simulink model "MotionLab"  (R2024a)
settings: Solver=VariableStepAuto  StartTime=0.0  StopTime=20  RelTol=1e-3  AbsTol=1e-3
values from neighbouring files (symbols this model uses):
  AmplitudeHeave = 0    [HMIVars.m]
  AmplitudePitch = 0    [HMIVars.m]
  AmplitudeRoll = 0    [HMIVars.m]
  AmplitudeSurge = 0    [HMIVars.m]
  AmplitudeSway = 0    [HMIVars.m]
  AmplitudeYaw = 0    [HMIVars.m]
  FrequencyHeave = 0    [HMIVars.m]
  FrequencyPitch = 0    [HMIVars.m]
  FrequencyRoll = 0    [HMIVars.m]
  FrequencySurge = 0    [HMIVars.m]
  FrequencySway = 0    [HMIVars.m]
  FrequencyYaw = 0    [HMIVars.m]
  OffsetHeave = 0    [HMIVars.m]
  OffsetPitch = 0    [HMIVars.m]
  OffsetRoll = 0    [HMIVars.m]
  OffsetSurge = 0    [HMIVars.m]
  OffsetSway = 0    [HMIVars.m]
  OffsetYaw = 0    [HMIVars.m]
  PhaseHeave = 0    [HMIVars.m]
  PhasePitch = 0    [HMIVars.m]
  PhaseRoll = 0    [HMIVars.m]
  PhaseSurge = 0    [HMIVars.m]
  PhaseSway = 0    [HMIVars.m]
  PhaseYaw = 0    [HMIVars.m]
undefined symbols (not defined in the file or in its folder): smiData, smiDataBig, smiDataBigTop, smiDataRobot, Var, X, Y, Z
libraries: sm_lib x438, nesl_utility x74
(part 14 of 14)

== system MotionLab/VHT eMotion-8000 Stewart Platform/UiA Stewart Platform/Top Platform/x3_134056_CARDAN_STEUN_stp_2_RIGID ==
  ReferenceFrame : sm_lib/Frames and Transforms/Reference Frame
  Solid : sm_lib/Body Elements/File Solid  ExtGeomFileName=.\CAD_Store\3-134056_CARDAN_STEUN.stp_Default_sldprt.STEP  UnitType=FromFile  ExtGeomFileUnits=m  StepReaderType=HEX  ExportConvexHullGeometry=off  InertiaType=Custom  BasedOnType=DensityFromFile  Density=1000  DensityUnits=kg/m^3  Mass=smiDataBig.Solid(7).mass  MassUnits=kg  CenterOfMass=smiDataBig.Solid(7).CoM  CenterOfMassUnits=mm  MomentsOfInertia=smiDataBig.Solid(7).MoI  MomentsOfInertiaUnits=kg*mm^2  ProductsOfInertia=smiDataBig.Solid(7).PoI  ProductsOfInertiaUnits=kg*mm^2  GraphicType=FromGeometry  MarkerShape=Sphere  MarkerSize=10  GraphicVisPropType=SimpleVisualProperties  GraphicDiffuseColor=smiDataBig.Solid(7).color  GraphicOpacity=smiDataBig.Solid(7).opacity  GraphicSpecularColor=[0.5 0.5 0.5 1.0]  GraphicAmbientColor=[0.15 0.15 0.15 1.0]  GraphicEmissiveColor=[0.0 0.0 0.0 1.0]  GraphicShininess=75  DoExposeReferenceFrame=on  SerializedFrames=<Frames><Frame><Id>Frame1</Id><Value><Name>F1</Name><Origin><Source>GeometricFeature</Source><FeatureName>cylindrical surface 89</FeatureName></Origin><PrimaryAxis><DefinedDirection>-Y</DefinedDirection><Source>ReferenceFrame</Source><SourceDirection>+Z</SourceDirection><FeatureName></FeatureName></PrimaryAxis><SecondaryAxis><DefinedDirection>+X</DefinedDirection><Source>ReferenceFrame</Source><SourceDirection>+X</SourceDirection><FeatureName></FeatureName></SecondaryAxis></Value></Frame><Frame><Id>Frame2</Id><Value><Name>F2</Name><Origin><Source>GeometricFeature</Source><FeatureName>cylindrical surface 83</FeatureName></Origin><PrimaryAxis><DefinedDirection>-Y</DefinedDirection><Source>ReferenceFrame</Source><SourceDirection>+Z</SourceDirection><FeatureName></FeatureName></PrimaryAxis><SecondaryAxis><DefinedDirection>+X</DefinedDirection><Source>ReferenceFrame</Source><SourceDirection>+X</SourceDirection><FeatureName></FeatureName></SecondaryAxis></Value></Frame><Frame><Id>Frame3</Id><Value><Name>F3</Name><Origin><Source>GeometricFeature</Source><FeatureName>planar surface 25</FeatureName></Origin><PrimaryAxis><DefinedDirection>+Z</DefinedDirection><Source>ReferenceFrame</Source><SourceDirection>+Z</SourceDirection><FeatureName></FeatureName></PrimaryAxis><SecondaryAxis><DefinedDirection>+X</DefinedDirection><Source>ReferenceFrame</Source><SourceDirection>+X</SourceDirection><FeatureName></FeatureName></SecondaryAxis></Value></Frame></Frames>
  F : PMIOPort  Side=Left
  F1 : PMIOPort  Port=2  Side=Right
  F2 : PMIOPort  Port=3  Side=Right
  connections:
  Solid/LConn1 -- F1/RConn1
  Solid/RConn2 -- ReferenceFrame/RConn1 -- F/RConn1
  Solid/LConn2 -- F2/RConn1

== system MotionLab/VHT eMotion-8000 Stewart Platform/UiA Stewart Platform/Top Platform/x3_134056_CARDAN_STEUN_stp_3_RIGID ==
  ReferenceFrame : sm_lib/Frames and Transforms/Reference Frame
  Solid : sm_lib/Body Elements/File Solid  ExtGeomFileName=.\CAD_Store\3-134056_CARDAN_STEUN.stp_Default_sldprt.STEP  UnitType=FromFile  ExtGeomFileUnits=m  StepReaderType=HEX  ExportConvexHullGeometry=off  InertiaType=Custom  BasedOnType=DensityFromFile  Density=1000  DensityUnits=kg/m^3  Mass=smiDataBig.Solid(7).mass  MassUnits=kg  CenterOfMass=smiDataBig.Solid(7).CoM  CenterOfMassUnits=mm  MomentsOfInertia=smiDataBig.Solid(7).MoI  MomentsOfInertiaUnits=kg*mm^2  ProductsOfInertia=smiDataBig.Solid(7).PoI  ProductsOfInertiaUnits=kg*mm^2  GraphicType=FromGeometry  MarkerShape=Sphere  MarkerSize=10  GraphicVisPropType=SimpleVisualProperties  GraphicDiffuseColor=smiDataBig.Solid(7).color  GraphicOpacity=smiDataBig.Solid(7).opacity  GraphicSpecularColor=[0.5 0.5 0.5 1.0]  GraphicAmbientColor=[0.15 0.15 0.15 1.0]  GraphicEmissiveColor=[0.0 0.0 0.0 1.0]  GraphicShininess=75  DoExposeReferenceFrame=on  SerializedFrames=<Frames><Frame><Id>Frame1</Id><Value><Name>F1</Name><Origin><Source>GeometricFeature</Source><FeatureName>cylindrical surface 89</FeatureName></Origin><PrimaryAxis><DefinedDirection>-Y</DefinedDirection><Source>ReferenceFrame</Source><SourceDirection>+Z</SourceDirection><FeatureName></FeatureName></PrimaryAxis><SecondaryAxis><DefinedDirection>+X</DefinedDirection><Source>ReferenceFrame</Source><SourceDirection>+X</SourceDirection><FeatureName></FeatureName></SecondaryAxis></Value></Frame><Frame><Id>Frame2</Id><Value><Name>F2</Name><Origin><Source>GeometricFeature</Source><FeatureName>cylindrical surface 83</FeatureName></Origin><PrimaryAxis><DefinedDirection>-Y</DefinedDirection><Source>ReferenceFrame</Source><SourceDirection>+Z</SourceDirection><FeatureName></FeatureName></PrimaryAxis><SecondaryAxis><DefinedDirection>+X</DefinedDirection><Source>ReferenceFrame</Source><SourceDirection>+X</SourceDirection><FeatureName></FeatureName></SecondaryAxis></Value></Frame><Frame><Id>Frame3</Id><Value><Name>F3</Name><Origin><Source>GeometricFeature</Source><FeatureName>planar surface 25</FeatureName></Origin><PrimaryAxis><DefinedDirection>+Z</DefinedDirection><Source>ReferenceFrame</Source><SourceDirection>+Z</SourceDirection><FeatureName></FeatureName></PrimaryAxis><SecondaryAxis><DefinedDirection>+X</DefinedDirection><Source>ReferenceFrame</Source><SourceDirection>+X</SourceDirection><FeatureName></FeatureName></SecondaryAxis></Value></Frame></Frames>
  F : PMIOPort  Side=Left
  F1 : PMIOPort  Port=2  Side=Right
  F2 : PMIOPort  Port=3  Side=Right
  connections:
  Solid/LConn2 -- F2/RConn1
  Solid/LConn1 -- F1/RConn1
  Solid/RConn2 -- ReferenceFrame/RConn1 -- F/RConn1

== system MotionLab/VHT eMotion-8000 Stewart Platform/UiA Stewart Platform/BaseFrame/x03_21_1320_ADM_Lower_Cardan_Baseplate_stp_1_RIGID/x03_21_1320_PDM_Base_Plate_stp_1_RIGID ==
  ReferenceFrame : sm_lib/Frames and Transforms/Reference Frame
  Solid : sm_lib/Body Elements/File Solid  ExtGeomFileName=.\CAD_Store\03-21-1320-PDM-Base Plate.stp_Default_sldprt.STEP  UnitType=FromFile  ExtGeomFileUnits=m  StepReaderType=HEX  ExportConvexHullGeometry=off  InertiaType=Custom  BasedOnType=DensityFromFile  Density=1000  DensityUnits=kg/m^3  Mass=smiDataBig.Solid(5).mass  MassUnits=kg  CenterOfMass=smiDataBig.Solid(5).CoM  CenterOfMassUnits=mm  MomentsOfInertia=smiDataBig.Solid(5).MoI  MomentsOfInertiaUnits=kg*mm^2  ProductsOfInertia=smiDataBig.Solid(5).PoI  ProductsOfInertiaUnits=kg*mm^2  GraphicType=FromGeometry  MarkerShape=Sphere  MarkerSize=10  GraphicVisPropType=SimpleVisualProperties  GraphicDiffuseColor=smiDataBig.Solid(5).color  GraphicOpacity=smiDataBig.Solid(5).opacity  GraphicSpecularColor=[0.5 0.5 0.5 1.0]  GraphicAmbientColor=[0.15 0.15 0.15 1.0]  GraphicEmissiveColor=[0.0 0.0 0.0 1.0]  GraphicShininess=75  DoExposeReferenceFrame=on  SerializedFrames=<Frames/>
  F : PMIOPort  Side=Left
  connections:
  ReferenceFrame/RConn1 -- Solid/RConn1 -- F/RConn1

== system MotionLab/VHT eMotion-8000 Stewart Platform/UiA Stewart Platform/BaseFrame/x03_21_1320_ADM_Lower_Cardan_Baseplate_stp_1_RIGID/x03_21_1320_PDM_Midplate_stp_1_RIGID ==
  ReferenceFrame : sm_lib/Frames and Transforms/Reference Frame
  Solid : sm_lib/Body Elements/File Solid  ExtGeomFileName=.\CAD_Store\03-21-1320-PDM-Midplate.stp_Default_sldprt.STEP  UnitType=FromFile  ExtGeomFileUnits=m  StepReaderType=HEX  ExportConvexHullGeometry=off  InertiaType=Custom  BasedOnType=DensityFromFile  Density=1000  DensityUnits=kg/m^3  Mass=smiDataBig.Solid(6).mass  MassUnits=kg  CenterOfMass=smiDataBig.Solid(6).CoM  CenterOfMassUnits=mm  MomentsOfInertia=smiDataBig.Solid(6).MoI  MomentsOfInertiaUnits=kg*mm^2  ProductsOfInertia=smiDataBig.Solid(6).PoI  ProductsOfInertiaUnits=kg*mm^2  GraphicType=FromGeometry  MarkerShape=Sphere  MarkerSize=10  GraphicVisPropType=SimpleVisualProperties  GraphicDiffuseColor=smiDataBig.Solid(6).color  GraphicOpacity=smiDataBig.Solid(6).opacity  GraphicSpecularColor=[0.5 0.5 0.5 1.0]  GraphicAmbientColor=[0.15 0.15 0.15 1.0]  GraphicEmissiveColor=[0.0 0.0 0.0 1.0]  GraphicShininess=75  DoExposeReferenceFrame=on  SerializedFrames=<Frames/>
  F : PMIOPort  Side=Left
  connections:
  ReferenceFrame/RConn1 -- Solid/RConn1 -- F/RConn1

== system MotionLab/VHT eMotion-8000 Stewart Platform/UiA Stewart Platform/BaseFrame/x03_21_1320_ADM_Lower_Cardan_Baseplate_stp_2_RIGID/x03_21_1320_PDM_Base_Plate_stp_1_RIGID ==
  ReferenceFrame : sm_lib/Frames and Transforms/Reference Frame
  Solid : sm_lib/Body Elements/File Solid  ExtGeomFileName=.\CAD_Store\03-21-1320-PDM-Base Plate.stp_Default_sldprt.STEP  UnitType=FromFile  ExtGeomFileUnits=m  StepReaderType=HEX  ExportConvexHullGeometry=off  InertiaType=Custom  BasedOnType=DensityFromFile  Density=1000  DensityUnits=kg/m^3  Mass=smiDataBig.Solid(5).mass  MassUnits=kg  CenterOfMass=smiDataBig.Solid(5).CoM  CenterOfMassUnits=mm  MomentsOfInertia=smiDataBig.Solid(5).MoI  MomentsOfInertiaUnits=kg*mm^2  ProductsOfInertia=smiDataBig.Solid(5).PoI  ProductsOfInertiaUnits=kg*mm^2  GraphicType=FromGeometry  MarkerShape=Sphere  MarkerSize=10  GraphicVisPropType=SimpleVisualProperties  GraphicDiffuseColor=smiDataBig.Solid(5).color  GraphicOpacity=smiDataBig.Solid(5).opacity  GraphicSpecularColor=[0.5 0.5 0.5 1.0]  GraphicAmbientColor=[0.15 0.15 0.15 1.0]  GraphicEmissiveColor=[0.0 0.0 0.0 1.0]  GraphicShininess=75  DoExposeReferenceFrame=on  SerializedFrames=<Frames/>
  F : PMIOPort  Side=Left
  connections:
  ReferenceFrame/RConn1 -- Solid/RConn1 -- F/RConn1

== system MotionLab/VHT eMotion-8000 Stewart Platform/UiA Stewart Platform/BaseFrame/x03_21_1320_ADM_Lower_Cardan_Baseplate_stp_2_RIGID/x03_21_1320_PDM_Midplate_stp_1_RIGID ==
  ReferenceFrame : sm_lib/Frames and Transforms/Reference Frame
  Solid : sm_lib/Body Elements/File Solid  ExtGeomFileName=.\CAD_Store\03-21-1320-PDM-Midplate.stp_Default_sldprt.STEP  UnitType=FromFile  ExtGeomFileUnits=m  StepReaderType=HEX  ExportConvexHullGeometry=off  InertiaType=Custom  BasedOnType=DensityFromFile  Density=1000  DensityUnits=kg/m^3  Mass=smiDataBig.Solid(6).mass  MassUnits=kg  CenterOfMass=smiDataBig.Solid(6).CoM  CenterOfMassUnits=mm  MomentsOfInertia=smiDataBig.Solid(6).MoI  MomentsOfInertiaUnits=kg*mm^2  ProductsOfInertia=smiDataBig.Solid(6).PoI  ProductsOfInertiaUnits=kg*mm^2  GraphicType=FromGeometry  MarkerShape=Sphere  MarkerSize=10  GraphicVisPropType=SimpleVisualProperties  GraphicDiffuseColor=smiDataBig.Solid(6).color  GraphicOpacity=smiDataBig.Solid(6).opacity  GraphicSpecularColor=[0.5 0.5 0.5 1.0]  GraphicAmbientColor=[0.15 0.15 0.15 1.0]  GraphicEmissiveColor=[0.0 0.0 0.0 1.0]  GraphicShininess=75  DoExposeReferenceFrame=on  SerializedFrames=<Frames/>
  F : PMIOPort  Side=Left
  connections:
  ReferenceFrame/RConn1 -- Solid/RConn1 -- F/RConn1

== system MotionLab/VHT eMotion-8000 Stewart Platform/UiA Stewart Platform/BaseFrame/x03_21_1320_ADM_Lower_Cardan_Baseplate_stp_3_RIGID/x03_21_1320_PDM_Base_Plate_stp_1_RIGID ==
  ReferenceFrame : sm_lib/Frames and Transforms/Reference Frame
  Solid : sm_lib/Body Elements/File Solid  ExtGeomFileName=.\CAD_Store\03-21-1320-PDM-Base Plate.stp_Default_sldprt.STEP  UnitType=FromFile  ExtGeomFileUnits=m  StepReaderType=HEX  ExportConvexHullGeometry=off  InertiaType=Custom  BasedOnType=DensityFromFile  Density=1000  DensityUnits=kg/m^3  Mass=smiDataBig.Solid(5).mass  MassUnits=kg  CenterOfMass=smiDataBig.Solid(5).CoM  CenterOfMassUnits=mm  MomentsOfInertia=smiDataBig.Solid(5).MoI  MomentsOfInertiaUnits=kg*mm^2  ProductsOfInertia=smiDataBig.Solid(5).PoI  ProductsOfInertiaUnits=kg*mm^2  GraphicType=FromGeometry  MarkerShape=Sphere  MarkerSize=10  GraphicVisPropType=SimpleVisualProperties  GraphicDiffuseColor=smiDataBig.Solid(5).color  GraphicOpacity=smiDataBig.Solid(5).opacity  GraphicSpecularColor=[0.5 0.5 0.5 1.0]  GraphicAmbientColor=[0.15 0.15 0.15 1.0]  GraphicEmissiveColor=[0.0 0.0 0.0 1.0]  GraphicShininess=75  DoExposeReferenceFrame=on  SerializedFrames=<Frames/>
  F : PMIOPort  Side=Left
  connections:
  ReferenceFrame/RConn1 -- Solid/RConn1 -- F/RConn1

== system MotionLab/VHT eMotion-8000 Stewart Platform/UiA Stewart Platform/BaseFrame/x03_21_1320_ADM_Lower_Cardan_Baseplate_stp_3_RIGID/x03_21_1320_PDM_Midplate_stp_1_RIGID ==
  ReferenceFrame : sm_lib/Frames and Transforms/Reference Frame
  Solid : sm_lib/Body Elements/File Solid  ExtGeomFileName=.\CAD_Store\03-21-1320-PDM-Midplate.stp_Default_sldprt.STEP  UnitType=FromFile  ExtGeomFileUnits=m  StepReaderType=HEX  ExportConvexHullGeometry=off  InertiaType=Custom  BasedOnType=DensityFromFile  Density=1000  DensityUnits=kg/m^3  Mass=smiDataBig.Solid(6).mass  MassUnits=kg  CenterOfMass=smiDataBig.Solid(6).CoM  CenterOfMassUnits=mm  MomentsOfInertia=smiDataBig.Solid(6).MoI  MomentsOfInertiaUnits=kg*mm^2  ProductsOfInertia=smiDataBig.Solid(6).PoI  ProductsOfInertiaUnits=kg*mm^2  GraphicType=FromGeometry  MarkerShape=Sphere  MarkerSize=10  GraphicVisPropType=SimpleVisualProperties  GraphicDiffuseColor=smiDataBig.Solid(6).color  GraphicOpacity=smiDataBig.Solid(6).opacity  GraphicSpecularColor=[0.5 0.5 0.5 1.0]  GraphicAmbientColor=[0.15 0.15 0.15 1.0]  GraphicEmissiveColor=[0.0 0.0 0.0 1.0]  GraphicShininess=75  DoExposeReferenceFrame=on  SerializedFrames=<Frames/>
  F : PMIOPort  Side=Left
  connections:
  ReferenceFrame/RConn1 -- Solid/RConn1 -- F/RConn1

== matlab function MotionLab/VHT eMotion-8000 Stewart Platform/UiA Stewart Platform/MATLAB Function ==
  data: R input; yaw output; pitch output; roll output
function [yaw, pitch, roll] = rotationMatrixToYPR(R)
    % Extract rotation matrix elements
    r11 = R(1,1); r12 = R(1,2); r13 = R(1,3);
    r21 = R(2,1); r22 = R(2,2); r23 = R(2,3);
    r31 = R(3,1); r32 = R(3,2); r33 = R(3,3);
    
    % Calculate yaw, pitch, and roll
    yaw = atan2(r21, r11);
    pitch = atan2(-r31, sqrt(r32^2 + r33^2));
    roll = atan2(r32, r33);
end

== matlab function MotionLab/VHT eMotion-1500 Stewart Platform/Motion Control System/MotionGen ==
  data: t input; motion output; R_top output; p_top output; AmplitudeSurge input; FrequencySurge input; PhaseSurge input; OffsetSurge input; AmplitudeSway input; FrequencySway input; PhaseSway input; OffsetSway input; AmplitudeHeave input; FrequencyHeave input; PhaseHeave input; OffsetHeave input; AmplitudeRoll input; FrequencyRoll input; PhaseRoll input; OffsetRoll input; AmplitudePitch input; FrequencyPitch input; PhasePitch input; OffsetPitch input; AmplitudeYaw input; FrequencyYaw input; PhaseYaw input; OffsetYaw input
function [motion,R_top,p_top] = platform_motion(t,AmplitudeSurge, FrequencySurge, PhaseSurge, OffsetSurge,AmplitudeSway, FrequencySway, PhaseSway, OffsetSway,AmplitudeHeave, FrequencyHeave, PhaseHeave, OffsetHeave,AmplitudeRoll, FrequencyRoll, PhaseRoll, OffsetRoll,AmplitudePitch, FrequencyPitch, PhasePitch, OffsetPitch,AmplitudeYaw, FrequencyYaw, PhaseYaw, OffsetYaw)
    % Define wave parameters for each degree of freedom
    % x, y, and z are translations (meters)
    % Roll, Pitch, and Yaw are rotations (radians)
    %Parameters, Amplitude, Frequency, Phase and Offset 
    % x (Surge) wave parameters
    x_params = [AmplitudeSurge, FrequencySurge, PhaseSurge, OffsetSurge];  
    % y (Sway) wave parameters
    y_params = [AmplitudeSway, FrequencySway, PhaseSway, OffsetSway];   
    % z (Heave) wave parameters
    z_params = [AmplitudeHeave, FrequencyHeave, PhaseHeave, OffsetHeave]; 
    % Roll wave parameters
    roll_params = [AmplitudeRoll, FrequencyRoll, PhaseRoll, OffsetRoll];  
    % Pitch wave parameters
    pitch_params = [AmplitudePitch, FrequencyPitch, PhasePitch, OffsetPitch]; 
    % Yaw wave parameters
    yaw_params = [AmplitudeYaw, FrequencyYaw, PhaseYaw, OffsetYaw]; 


    %Parameters, Amplitude, Frequency, Phase and Offset 
    % x (Surge) wave parameters
    %x_params = [0.05, 0.05, 0, 0];  
    % y (Sway) wave parameters
    %y_params = [0.05, 0.05, pi/2, 0];   
    % z (Heave) wave parameters
    %z_params = [0.2; 0.1; 0; 1.55]; 
    % Roll wave parameters
   % roll_params = [deg2rad(3), 0.07, 0, 0];  
    % Pitch wave parameters
   % pitch_params = [deg2rad(3), 0.05, pi/2, 0]; 
    % Yaw wave parameters
   % yaw_params = [deg2rad(2), 0.05, pi/2, 0]; 
    

    % Calculate the motion for each degree of freedom
    x = x_params(1) * sin(2 * pi * x_params(2) * t + x_params(3)) + x_params(4);
    y = y_params(1) * sin(2 * pi * y_params(2) * t + y_params(3)) + y_params(4);
    z = z_params(1) * sin(2 * pi * z_params(2) * t + z_params(3)) + z_params(4) + 2.88;
    roll = roll_params(1) * sin(2 * pi * roll_params(2) * t + roll_params(3)) + roll_params(4);
    pitch = pitch_params(1) * sin(2 * pi * pitch_params(2) * t + pitch_params(3)) + pitch_params(4);
    yaw = yaw_params(1) * sin(2 * pi * yaw_params(2) * t + yaw_params(3)) + yaw_params(4);

    % Combine all motions into a single output vector
    motion = [x; y; z; roll; pitch; yaw];

    % Translational components
    p_top_x = x;  % X position
    p_top_y = y;  % Y position
    p_top_z = z;  % Z position

    % Rotational components
    theta_x = roll;  % Rotation about X axis
    theta_y = pitch;  % Rotation about Y axis
    theta_z = yaw;  % Rotation about Z axis

    % Position vector
    p_top = [p_top_x; p_top_y; p_top_z];

    % Rotation matrix
    eul = [theta_z, theta_y, theta_x];
    R_top = eul2rotm(eul);  % Euler angles to rotation matrix

end

== matlab function MotionLab/VHT eMotion-8000 Stewart Platform/Inverse Kinematics/InvKin ==
  data: RotBig input; wBig input; posBig input; f output; velBig input; g output
function [f,g] = fcn(RotBig,wBig,posBig,velBig)
%Static Variables
Lmin = 2.68687; %Joint to joint length fully compressed
%A is ground, B is Top
p_AibC1 = [1.35616,-2.12033,0.25]';
p_AibC2 = [1.15818,-2.23463,0.25]';
p_AibC3 = [-2.51434,-0.1143,0.25]';
p_AibC4 = [-2.51343,0.1143,0.25]';
p_AibC5 = [1.15818,2.23463,0.25]';
p_AibC6 = [1.35616,2.12033,0.25]';

p_BitC1 = [2.11178,-0.1143,0.00002]'; 
p_BitC2 = [-0.9561,-1.88787,0.00002]';
p_BitC3 = [-1.15487,-1.7717,0.00002]';
p_BitC4 = [-1.15487,1.7717,0.00002]';
p_BitC5 = [-0.9569,1.886,0.00002]';
p_BitC6 = [2.11178,0.1143,0.00002]';

p_tb = [posBig(1);posBig(2); posBig(3)];
R = RotBig;
w_tb = wBig';
pdot_tb = velBig;

%CYLINDER 1
p_Bib1 = p_tb + R*p_BitC1;
p_BAib1 = p_Bib1 - p_AibC1;
Li1 = norm(p_BAib1);
ui1 = p_BAib1/Li1;
qi1 = Li1 - Lmin; 
qdot_i1 = ui1'*pdot_tb + cross(w_tb, R*p_BitC1)*ui1;
Jinv1 = [ui1,(R*p_BitC1*ui1')]; 


%CYLINDER 2:
p_Bib2 = p_tb + R*p_BitC2;
p_BAib2 = p_Bib2 - p_AibC2;
Li2 = norm(p_BAib2);
ui2 = p_BAib2/Li2;
qi2 = Li2 - Lmin; 
qdot_i2 = ui2' * pdot_tb + cross(w_tb, R*p_BitC2)*ui2; 
Jinv2 = [ui2,(R*p_BitC2*ui2')];

%CYLINDER 3:
p_Bib3 = p_tb + R*p_BitC3;
p_BAib3 = p_Bib3 - p_AibC3;
Li3 = norm(p_BAib3);
ui3 = p_BAib3/Li3;
qi3 = Li3 - Lmin;
qdot_i3 = ui3' * pdot_tb + cross(w_tb,R*p_BitC3)*ui3; 
Jinv3 = [ui3,(R*p_BitC3*ui3')]; 

%CYLINDER 4:
p_Bib4 = p_tb + R*p_BitC4;
p_BAib4 = p_Bib4 - p_AibC4;
Li4 = norm(p_BAib4);
ui4 = p_BAib4/Li4;
qi4 = Li4 - Lmin;
qdot_i4 = ui4' * pdot_tb + cross(w_tb,R*p_BitC4)*ui4; 
Jinv4 = [ui4,(R*p_BitC4*ui4')]; 


%CYLINDER 5:
p_Bib5 = p_tb + R*p_BitC5;
p_BAib5 = p_Bib5 - p_AibC5;
Li5 = norm(p_BAib5);
ui5 = p_BAib5/Li5;
qi5 = Li5 - Lmin; 
qdot_i5 = ui5' * pdot_tb + cross(w_tb,R*p_BitC5)*ui5; 
Jinv5 = [ui5,(R*p_BitC5*ui5')]; 

%CYLINDER 6:
p_Bib6 = p_tb + R*p_BitC6;
p_BAib6 = p_Bib6 - p_AibC6;
Li6 = norm(p_BAib6);
ui6 = p_BAib6/Li6;
qi6 = Li6 - Lmin; 
qdot_i6 = ui6' * pdot_tb + cross(w_tb,R*p_BitC6)*ui6; 
Jinv6 = [ui6,(R*p_BitC6*ui6')]; 

%Desired 6DOF vel of top platform to cyl joint vel:
%Jinv = [Jinv1;Jinv2;Jinv3;Jinv4;Jinv5;Jinv6];
%qdot = Jinv*[pdot_tb;w_tb]

f = [qi1,qi2,qi3,qi4,qi5,qi6]; 
g = [qdot_i1, qdot_i2, qdot_i3, qdot_i4, qdot_i5, qdot_i6];

== matlab function MotionLab/VHT eMotion-1500 Stewart Platform/Inverse Kinematics1/MATLAB Function ==
  data: Rot input; w input; pos input; f output; vel input; g output
function [f,g] = fcn(Rot,w,pos,vel)

%Static Variables
Lmin = 1.456215; %Joint to joint length currenctly(1.456215m)

p_AibC1 = [0.70416,-1.02102,0.11258]';
p_AibC2 = [0.53215,-1.12033,0.11258]';
p_AibC3 = [-1.23631,-0.09931,0.11258]';
p_AibC4 = [-1.23631,0.09931,0.11258]';
p_AibC5 = [0.53215,1.12033,0.11258]';
p_AibC6 = [0.70416,1.02102,0.11258]';

p_BitC1 = [0.95000,-0.09000,0]';
p_BitC2 = [-0.39706,-0.86772,0]';
p_BitC3 = [-0.55294,-0.77772,0]';
p_BitC4 = [-0.55294,0.77772,0]';
p_BitC5 = [-0.39706,0.86772,0]';
p_BitC6 = [0.95000,0.09000,0]';

p_tb = [pos(1);pos(2); pos(3)];
R = Rot;
w_tb = w';
pdot_tb = vel;

%CYLINDER 1
p_Bib1 = p_tb + R*p_BitC1;
p_BAib1 = p_Bib1 - p_AibC1;
Li1 = norm(p_BAib1);
ui1 = p_BAib1/Li1;
qi1 = Li1 - Lmin; 
%pdot_Bib1 = pdot_tb + w_tb*R*p_BitC1;
qdot_i1 = ui1'*pdot_tb + cross(w_tb, R*p_BitC1)*ui1;
Jinv1 = [ui1,(R*p_BitC1*ui1')]; 


%CYLINDER 2:
p_Bib2 = p_tb + R*p_BitC2;
p_BAib2 = p_Bib2 - p_AibC2;
Li2 = norm(p_BAib2);
ui2 = p_BAib2/Li2;
qi2 = Li2 - Lmin; 
%pdot_Bib2 = pdot_tb + w_tb*R*p_BitC2;
qdot_i2 = ui2' * pdot_tb + cross(w_tb, R*p_BitC2)*ui2; 
Jinv2 = [ui2,(R*p_BitC2*ui2')];

%CYLINDER 3:
p_Bib3 = p_tb + R*p_BitC3;
p_BAib3 = p_Bib3 - p_AibC3;
Li3 = norm(p_BAib3);
ui3 = p_BAib3/Li3;
qi3 = Li3 - Lmin;
%pdot_Bib3 = pdot_tb + w_tb*R*p_BitC3;
qdot_i3 = ui3' * pdot_tb + cross(w_tb,R*p_BitC3)*ui3; 
Jinv3 = [ui3,(R*p_BitC3*ui3')]; 

%CYLINDER 4:
p_Bib4 = p_tb + R*p_BitC4;
p_BAib4 = p_Bib4 - p_AibC4;
Li4 = norm(p_BAib4);
ui4 = p_BAib4/Li4;
qi4 = Li4 - Lmin;
%pdot_Bib4 = pdot_tb + w_tb*R*p_BitC4;
qdot_i4 = ui4' * pdot_tb + cross(w_tb,R*p_BitC4)*ui4; 
Jinv4 = [ui4,(R*p_BitC4*ui4')]; 


%CYLINDER 5:
p_Bib5 = p_tb + R*p_BitC5;
p_BAib5 = p_Bib5 - p_AibC5;
Li5 = norm(p_BAib5);
ui5 = p_BAib5/Li5;
qi5 = Li5 - Lmin; 
%pdot_Bib5 = pdot_tb + w_tb*R*p_BitC5;
qdot_i5 = ui5' * pdot_tb + cross(w_tb,R*p_BitC5)*ui5; 
Jinv5 = [ui5,(R*p_BitC5*ui5')]; 

%CYLINDER 6:
p_Bib6 = p_tb + R*p_BitC6;
p_BAib6 = p_Bib6 - p_AibC6;
Li6 = norm(p_BAib6);
ui6 = p_BAib6/Li6;
qi6 = Li6 - Lmin; 
%pdot_Bib6 = pdot_tb + w_tb*R*p_BitC6;
qdot_i6 = ui6' * pdot_tb + cross(w_tb,R*p_BitC6)*ui6; 
Jinv6 = [ui6,(R*p_BitC6*ui6')]; 

%Desired 6DOF vel of top platform to cyl joint vel:
Jinv = [Jinv1;Jinv2;Jinv3;Jinv4;Jinv5;Jinv6];
%pdot_tb_des = [x,y,z; yaw,pitch,roll] 

f = [qi1,qi2,qi3,qi4,qi5,qi6]; 
g = [qdot_i1, qdot_i2, qdot_i3, qdot_i4, qdot_i5, qdot_i6];

== matlab function MotionLab/VHT eMotion-8000 Stewart Platform/Motion Control System/MotionGen ==
  data: t input; motion output; R_top output; p_top output; AmplitudeSurge input; FrequencySurge input; PhaseSurge input; OffsetSurge input; AmplitudeSway input; FrequencySway input; PhaseSway input; OffsetSway input; AmplitudeHeave input; FrequencyHeave input; PhaseHeave input; OffsetHeave input; AmplitudeRoll input; FrequencyRoll input; PhaseRoll input; OffsetRoll input; AmplitudePitch input; FrequencyPitch input; PhasePitch input; OffsetPitch input; AmplitudeYaw input; FrequencyYaw input; PhaseYaw input; OffsetYaw input
function [motion,R_top,p_top] = platform_motion(t,AmplitudeSurge, FrequencySurge, PhaseSurge, OffsetSurge,AmplitudeSway, FrequencySway, PhaseSway, OffsetSway,AmplitudeHeave, FrequencyHeave, PhaseHeave, OffsetHeave,AmplitudeRoll, FrequencyRoll, PhaseRoll, OffsetRoll,AmplitudePitch, FrequencyPitch, PhasePitch, OffsetPitch,AmplitudeYaw, FrequencyYaw, PhaseYaw, OffsetYaw)
    % Define wave parameters for each degree of freedom
    % x, y, and z are translations (meters)
    % Roll, Pitch, and Yaw are rotations (radians)
    %Parameters, Amplitude, Frequency, Phase and Offset 
    % x (Surge) wave parameters
    x_params = [AmplitudeSurge, FrequencySurge, PhaseSurge, OffsetSurge];  
    % y (Sway) wave parameters
    y_params = [AmplitudeSway, FrequencySway, PhaseSway, OffsetSway];   
    % z (Heave) wave parameters
    z_params = [AmplitudeHeave, FrequencyHeave, PhaseHeave, OffsetHeave]; 
    % Roll wave parameters
    roll_params = [AmplitudeRoll, FrequencyRoll, PhaseRoll, OffsetRoll];  
    % Pitch wave parameters
    pitch_params = [AmplitudePitch, FrequencyPitch, PhasePitch, OffsetPitch]; 
    % Yaw wave parameters
    yaw_params = [AmplitudeYaw, FrequencyYaw, PhaseYaw, OffsetYaw]; 

    % Calculate the motion for each degree of freedom
    x = x_params(1) * sin(2 * pi * x_params(2) * t + x_params(3)) + x_params(4);
    y = y_params(1) * sin(2 * pi * y_params(2) * t + y_params(3)) + y_params(4);
    z = z_params(1) * sin(2 * pi * z_params(2) * t + z_params(3)) + z_params(4) + 2.88;
    roll = roll_params(1) * sin(2 * pi * roll_params(2) * t + roll_params(3)) + roll_params(4);
    pitch = pitch_params(1) * sin(2 * pi * pitch_params(2) * t + pitch_params(3)) + pitch_params(4);
    yaw = yaw_params(1) * sin(2 * pi * yaw_params(2) * t + yaw_params(3)) + yaw_params(4);

    % Combine all motions into a single output vector
    motion = [x; y; z; roll; pitch; yaw];

    % Translational components
    p_top_x = x;  % X position
    p_top_y = y;  % Y position
    p_top_z = z;  % Z position

    % Rotational components
    theta_x = roll;  % Rotation about X axis
    theta_y = pitch;  % Rotation about Y axis
    theta_z = yaw;  % Rotation about Z axis

    % Position vector
    p_top = [p_top_x; p_top_y; p_top_z];

    % Rotation matrix
    eul = [theta_z, theta_y, theta_x];
    R_top = eul2rotm(eul);  % Euler angles to rotation matrix

end
